simulink model "ScriptDemo"  (R2022b)
settings: configuration reference "TmVcThermal_Configuration_sub" (kept outside this file)
undefined symbols (not defined in the file or in its folder): aaaa, bbbb, cTmComprCtrl_D_u8HvacFlowTable_db, cTmComprCtrl_D_u8HvacFlowTable_sw, cTmComprCtrl_n_i16ChillCmpIMax, cTmComprCtrl_n_i16ChillCmpIMin, cTmComprCtrl_n_i16ChillCmpIMin666, cTmComprCtrl_n_i16ChillCmpPMax, cTmComprCtrl_n_i16ChillCmpPMin, cTmComprCtrl_n_i16CmpChillCoolRpmKiMax, cTmComprCtrl_n_i16CmpChillCoolRpmKiMin, cTmComprCtrl_n_i16CmpChillCoolRpmKpMax, cTmComprCtrl_n_i16CmpChillCoolRpmKpMin, cTmComprCtrl_n_i16CmpCoolRpmKiMax, cTmComprCtrl_n_i16CmpCoolRpmKiMin, cTmComprCtrl_n_i16CmpCoolRpmKpMax, cTmComprCtrl_n_i16CmpCoolRpmKpMin, cTmComprCtrl_n_i16SM4CmpHeatKiMax, cTmComprCtrl_n_i16SM4CmpHeatKiMin, cTmComprCtrl_n_i16SM4CmpHeatKpMax, cTmComprCtrl_n_i16SM4CmpHeatKpMin, cTmComprCtrl_n_i16SM5CmpHeatKiMax, cTmComprCtrl_n_i16SM5CmpHeatKiMin, cTmComprCtrl_n_i16SM5CmpHeatKpMax, cTmComprCtrl_n_i16SM5CmpHeatKpMin, cTmComprCtrl_n_i16SM6CmpHeatKiMax, cTmComprCtrl_n_i16SM6CmpHeatKiMin, cTmComprCtrl_n_i16SM6CmpHeatKpMax, cTmComprCtrl_n_i16SM6CmpHeatKpMin, cTmComprCtrl_n_u16CmpMaxSpdFanFltLimt, cTmComprCtrl_n_u16CmpMaxSpdLoSidePFltLimt, cTmComprCtrl_n_u16CmpMaxSpdSensorFltLimt, cTmComprCtrl_n_u16CompMinRpm, cTmComprCtrl_n_u16CompRpmIncThres, cTmComprCtrl_t_u16BattCooltFFPeriod, cTmComprCtrl_t_u16BattCooltPIPeriod, cTmComprCtrl_t_u16CmpCoolFFPeriod, cTmComprCtrl_t_u16CmpCoolPIPeriod, cTmComprCtrl_t_u16CoolCmpChillFFPeriod, cTmComprCtrl_t_u16CoolCmpChillPIPeriod, cTmComprCtrl_t_u16SM4CmpHeatFFPeriod, cTmComprCtrl_t_u16SM4CmpHeatPIPeriod, cTmComprCtrl_t_u16SM5CmpHeatFFPeriod, cTmComprCtrl_t_u16SM5CmpHeatPIPeriod, cTmComprCtrl_t_u16SM6CmpHeatFFPeriod, cTmComprCtrl_t_u16SM6CmpHeatPIPeriod, cTmComprCtrl_Te_EvapClearInteg, cTmComprCtrl_Te_i16HpReqTempSaturoffset, cTmComprCtrl_Te_i16SatLpReplaceDiff, cTmComprCtrl_Te_i16SM3BatDiffStartEvapDecOffset, cTmComprCtrl_Te_i16SM3EvapLo, cTmComprCtrl_Te_i16SM3TBatDiffEntEvapDecOffset, cTmComprCtrl_Te_i16SM3TBatDiffEntEvapDecOffsetQuit, cTmComprCtrl_Te_s32ErrCmpChillPIContinueCoolH, cTmComprCtrl_Te_s32ErrCmpChillPIContinueCoolL, cTmComprCtrl_Te_s32ErrCmpPIContinueChillH, cTmComprCtrl_Te_s32ErrCmpPIContinueChillL, cTmComprCtrl_Te_s32ErrCmpPIContinueCoolH, cTmComprCtrl_Te_s32ErrCmpPIContinueCoolL, cTmComprCtrl_Te_s32ErrCmpPIContinueHeatH ... (+398)
libraries: simulink x846, PCMULib x711, simulink_need_slupdate x4
(part 29 of 49)

== system ScriptDemo/Create/createMerge/After/SM3SM23/ID26262_SM3FF ==
  note: 0704：这里为什么用误差来查表？
  sTmSigProces_Te_s32EvapFanReqRamp : Inport  OutDataTypeStr=single
  sTmIn_D_u8DCChrgSt : Inport  Port=2  OutDataTypeStr=uint8
  sTmIn_Te_s32BattHv : Inport  Port=3  OutDataTypeStr=single
  sTmIn_X_s32ClimtRcirc : Inport  Port=4  OutDataTypeStr=single
  sTmComprCtrl_D_u8HvacFlowLevel : Inport  Port=5  OutDataTypeStr=uint8
  sTmSigProces_D_u8HvBattCoolgReq : Inport  Port=6  OutDataTypeStr=uint8
  xTmComprCtrl_B_CompOnReqCompOn : Inport  Port=7  OutDataTypeStr=boolean
  sTmIn_D_u8HeatPump : Inport  Port=8  OutDataTypeStr=uint8
  1-D Lookup Table1 : Lookup_n-D  NumberOfTableDimensions=1  BreakpointsForDimension1=tTmComprCtrl_n_s32Kcmp_X  BreakpointsForDimension1DataTypeStr=Inherit: Inherit from 'Breakpoint data'  Table=tTmComprCtrl_n_s32Kcmp  TableDataTypeStr=Inherit: Inherit from 'Table data'  ExtrapMethod=Clip  InternalRulePriority=Speed  OutDataTypeStr=Inherit: Inherit via back propagation  RndMeth=Simplest  InputSameDT=off
  1-D Lookup Table2 : Lookup_n-D  NumberOfTableDimensions=1  BreakpointsForDimension1=tTmComprCtrl_n_s32KChill_X  BreakpointsForDimension1DataTypeStr=Inherit: Inherit from 'Breakpoint data'  Table=tTmComprCtrl_n_s32KChill  TableDataTypeStr=Inherit: Inherit from 'Table data'  ExtrapMethod=Clip  InternalRulePriority=Speed  OutDataTypeStr=Inherit: Inherit via back propagation  RndMeth=Simplest  InputSameDT=off
  Add : Sum  OutDataTypeStr=uint16
  From7 : From  Commented=on  GotoTag=sTmIn_Te_s32HvBattCooltTReq
  Product : Product
  Product1 : Product
  SM1FFEnable : Subsystem
  SM2FFEnable : Subsystem
  SM3SM1FF : Subsystem
  SM3SM2FF : Subsystem
  SM3FF : Outport
  wires:
  [sTmIn_Te_s32BattHv] -> 1-D Lookup Table2/1
  1-D Lookup Table1/1 -> Product1/1  "Kcmp"
  1-D Lookup Table2/1 -> Product/2  "KChill"
  [sTmSigProces_Te_s32TAmb] -> 1-D Lookup Table1/1
  Product/1 -> Add/1
  [SM1FF] -> Product/1
  Product1/1 -> Add/2
  [SM2FF] -> Product1/2
  Add/1 -> SM3FF/1
  ? -> [sTmIn_Te_s32HvBattCooltTReq]
  sTmSigProces_Te_s32EvapFanReqRamp/1 -> [sTmSigProces_Te_s32EvapFanReqRamp]
  sTmIn_D_u8DCChrgSt/1 -> [sTmIn_D_u8DCChrgSt]
  ? -> [sTmSigProces_Te_s32TAmb]
  sTmIn_Te_s32BattHv/1 -> [sTmIn_Te_s32BattHv]
  sTmIn_X_s32ClimtRcirc/1 -> [sTmIn_X_s32ClimtRcirc]
  sTmComprCtrl_D_u8HvacFlowLevel/1 -> [sTmComprCtrl_D_u8HvacFlowLevel]
  sTmSigProces_D_u8HvBattCoolgReq/1 -> [sTmSigProces_D_u8HvBattCoolgReq]
  SM1FFEnable/1(SM1FFEnable_B_SM1FFEnable) -> [SM1FFEnable_B_SM1FFEnable]
  [xTmComprCtrl_B_CompOnReqCompOn] -> SM1FFEnable/1(xTmComprCtrl_B_CompOnReqCompOn)
  [SM1FFEnable_B_SM1FFEnable] -> SM3SM1FF/Enable
  [sTmSigProces_D_u8HvBattCoolgReq] -> SM3SM1FF/2(sTmSigProces_D_u8HvBattCoolgReq)
  [sTmIn_D_u8DCChrgSt] -> SM3SM1FF/1(sTmIn_D_u8DCChrgSt)
  [sTmIn_Te_s32HvBattCooltTReq] -> ?
  [SM2FFEnable_B_SM2FFEnable] -> SM3SM2FF/Enable
  [xTmComprCtrl_B_CompOnReqCompOn] -> SM2FFEnable/1(xTmComprCtrl_B_CompOnReqCompOn)
  SM2FFEnable/1(SM2FFEnable_B_SM2FFEnable) -> [SM2FFEnable_B_SM2FFEnable]
  SM3SM1FF/1(SM1FF) -> [SM1FF]  "rTmComprCtrl_n_u16ComprRpmFFSM3SM1"
  xTmComprCtrl_B_CompOnReqCompOn/1 -> [xTmComprCtrl_B_CompOnReqCompOn]
  [sTmSigProces_Te_s32TAmb] -> ?
  SM3SM2FF/1(SM2FF) -> [SM2FF]  "rTmComprCtrl_n_u16ComprRpmFFSM3SM2"
  [sTmSigProces_Te_s32EvapFanReqRamp] -> SM3SM2FF/1(sTmSigProces_Te_s32EvapFanReqRamp)
  [sTmSigProces_Te_s32TAmb] -> ?
  [sTmIn_X_s32ClimtRcirc] -> SM3SM2FF/2(sTmIn_X_s32ClimtRcirc)
  [sTmComprCtrl_D_u8HvacFlowLevel] -> SM3SM2FF/3(sTmComprCtrl_D_u8HvacFlowLevel)
  [sTmIn_D_u8HeatPump] -> SM3SM2FF/4(sTmIn_D_u8HeatPump)
  sTmIn_D_u8HeatPump/1 -> [sTmIn_D_u8HeatPump]
  [sTmIn_D_u8HeatPump] -> SM3SM1FF/3(sTmIn_D_u8HeatPump)

== system ScriptDemo/Create/createMerge/After/SM3SM23/ID26263_SM3Error ==
  note: 非热泵
  note: 1: 非热泵
      | 2：热泵
  note: 热泵
  sTmSigProces_Te_s32EvapFanReqRamp : Inport  OutDataTypeStr=single
  sTmIn_D_u8HeatPump : Inport  Port=2  OutDataTypeStr=uint8
  sTmSigProces_D_u8HvBattCoolgReq : Inport  Port=3  OutDataTypeStr=uint8
  sTmSigProces_Te_s32EvapFanFilter : Inport  Port=4  OutDataTypeStr=single
  xTmComprCtrl_B_ModeChanged : Inport  Port=5  OutDataTypeStr=boolean
  Compare To Constant1 : simulink/Logic and Bit Operations/Compare To Constant  relop===  const=2  OutDataTypeStr=boolean
  SM3HPErr : Subsystem
  SM3NHPErr : Subsystem
  Switch : Switch  Criteria=u2 ~= 0  SaturateOnIntegerOverflow=off  InputSameDT=off
  rTmComprCtrl_Te_s32TempError : Outport
  wires:
  Compare To Constant1/1 -> Switch/2
  [sTmIn_D_u8HeatPump] -> Compare To Constant1/1
  Switch/1 -> rTmComprCtrl_Te_s32TempError/1
  SM3NHPErr/1(SM3NHPErr_Te_s32Error) -> Switch/3
  SM3HPErr/1(SM3HPErr_Te_s32Error) -> Switch/1
  [sTmSigProces_Te_s32EvapFanReqRamp] -> SM3HPErr/1(sTmSigProces_Te_s32EvapFanReqRamp)
  [sTmIn_Te_s32HvBattCooltTReq] -> ?
  [sTmSigProces_Te_s32EvapFanFilter] -> SM3HPErr/2(sTmSigProces_Te_s32EvapFanFilter)
  [sTmSigProces_Te_s32HvBattCooltTFilter] -> ?
  [sTmSigProces_Te_s32EvapFanReqRamp] -> SM3NHPErr/1(sTmSigProces_Te_s32EvapFanReqRamp)
  [sTmIn_Te_s32HvBattCooltTReq] -> ?
  [sTmSigProces_D_u8HvBattCoolgReq] -> SM3NHPErr/2(sTmSigProces_D_u8HvBattCoolgReq)
  [sTmSigProces_Te_s32EvapFanFilter] -> SM3NHPErr/3(sTmSigProces_Te_s32EvapFanFilter)
  [sTmSigProces_Te_s32HvBattCooltTFilter] -> ?
  sTmSigProces_Te_s32EvapFanReqRamp/1 -> [sTmSigProces_Te_s32EvapFanReqRamp]
  sTmIn_D_u8HeatPump/1 -> [sTmIn_D_u8HeatPump]
  ? -> [sTmIn_Te_s32HvBattCooltTReq]
  sTmSigProces_D_u8HvBattCoolgReq/1 -> [sTmSigProces_D_u8HvBattCoolgReq]
  sTmSigProces_Te_s32EvapFanFilter/1 -> [sTmSigProces_Te_s32EvapFanFilter]
  ? -> [sTmSigProces_Te_s32HvBattCooltTFilter]
  [xTmComprCtrl_B_ModeChanged] -> SM3HPErr/3(xTmComprCtrl_B_ModeChanged)
  xTmComprCtrl_B_ModeChanged/1 -> [xTmComprCtrl_B_ModeChanged]

== system ScriptDemo/Create/createMerge/After/SM3SM23/SM3SM1Error ==
  "NegAndPosCheck " : Subsystem  AncestorBlock=CustomLib/TempNegAndPosCheck
  Terminator : Terminator
  rTmComprCtrl_Te_s32TempError : Outport  OutDataTypeStr=single
  wires:
  ? -> "NegAndPosCheck "/2(Acture)
  "NegAndPosCheck "/2(Dvt_PosFlag) -> Terminator/1
  ? -> "NegAndPosCheck "/1(SetPoint)
  "NegAndPosCheck "/1(Dvt) -> rTmComprCtrl_Te_s32TempError/1

== system ScriptDemo/Create/createMerge/After/SM3SM23/SM3SM2Error ==
  note: 控制对象为低压饱和温度
  note: 控制对象为蒸发器温度滤波值
  sTmSigProces_Te_s32EvapFanReqRamp : Inport  OutDataTypeStr=single
  sTmDiag_D_u8TeEvapFltSt : Inport  Port=2  OutDataTypeStr=uint8
  sTmSigProces_Te_s32EvapFanFilter : Inport  Port=3  OutDataTypeStr=single
  sTmSigProces_Te_s32SatLp : Inport  Port=4  OutDataTypeStr=single
  yTmRefriModeMgr_B_CoolOCRMode : Inport  Port=5  OutDataTypeStr=boolean
  Add : Sum  Inputs=+-  OutDataTypeStr=single
  Compare To Constant : simulink/Logic and Bit Operations/Compare To Constant  relop===  const=1  OutDataTypeStr=boolean
  Constant : Constant  Value=3  OutDataTypeStr=single
  Constant2 : Constant  Value=cTmComprCtrl_Te_i16SatLpReplaceDiff  OutDataTypeStr=int16
  NegAndPosCheck 1 : Subsystem  AncestorBlock=CustomLib/TempNegAndPosCheck
  Saturation1 : Saturate  UpperLimit=12  LowerLimit=3
  Switch1 : Switch  Criteria=u2 ~= 0  SaturateOnIntegerOverflow=off  InputSameDT=off
  Switch2 : Switch  Criteria=u2 ~= 0  SaturateOnIntegerOverflow=off  InputSameDT=off
  Terminator : Terminator
  rTmComprCtrl_Te_s32TempError : Outport
  wires:
  [sTmDiag_D_u8TeEvapFltSt] -> Switch1/2
  [sTmSigProces_Te_s32SatLp] -> Add/1
  Constant2/1 -> Add/2
  Switch2/1 -> Saturation1/1
  NegAndPosCheck 1/2(Dvt_PosFlag) -> Terminator/1
  NegAndPosCheck 1/1(Dvt) -> rTmComprCtrl_Te_s32TempError/1
  Add/1 -> Switch1/1
  Saturation1/1 -> NegAndPosCheck 1/1(SetPoint)
  sTmSigProces_Te_s32EvapFanReqRamp/1 -> [sTmSigProces_Te_s32EvapFanReqRamp]  "sTmSigProces_Te_s32EvapFanReqRamp"
  sTmDiag_D_u8TeEvapFltSt/1 -> [sTmDiag_D_u8TeEvapFltSt]  "sTmDiag_D_u8TeEvapFltSt"
  sTmSigProces_Te_s32EvapFanFilter/1 -> [sTmSigProces_Te_s32EvapFanFilter]  "sTmSigProces_Te_s32EvapFanFilter"
  sTmSigProces_Te_s32SatLp/1 -> [sTmSigProces_Te_s32SatLp]  "sTmSigProces_Te_s32SatLp"
  [yTmRefriModeMgr_B_CoolOCRMode] -> Compare To Constant/1
  Compare To Constant/1 -> Switch2/2
  Constant/1 -> Switch2/1
  yTmRefriModeMgr_B_CoolOCRMode/1 -> [yTmRefriModeMgr_B_CoolOCRMode]  "yTmRefriModeMgr_B_CoolOCRMode"
  [sTmSigProces_Te_s32EvapFanReqRamp] -> Switch2/3
  [sTmSigProces_Te_s32EvapFanFilter] -> Switch1/3
  Switch1/1 -> NegAndPosCheck 1/2(Acture)

== system ScriptDemo/Create/createMerge/After/SM3SM23/SM3_Ki ==
  note: 等级1或2
  note: 等级3
  SM1Error : Inport
  SM2Error : Inport  Port=2
  sTmIn_D_u8DCChrgSt : Inport  Port=3  OutDataTypeStr=uint8
  sTmIn_D_u8HeatPump : Inport  Port=4  OutDataTypeStr=uint8
  sTmIn_X_s32ClimtRcirc : Inport  Port=5  OutDataTypeStr=single
  sTmComprCtrl_D_u8HvacFlowLevel : Inport  Port=6  OutDataTypeStr=uint8
  sTmSigProces_D_u8BattThermReq : Inport  Port=7  OutDataTypeStr=uint8
  sTmSigProces_D_u8HvBattCoolgReq : Inport  Port=8  OutDataTypeStr=uint8
  Add : Sum
  Add1 : Sum
  Compare To Constant : simulink/Logic and Bit Operations/Compare To Constant  relop===  const=3  OutDataTypeStr=boolean
  SM1Ki : Subsystem
  SM2Ki : Subsystem
  SM3SM1LikeKi : Subsystem
  SM3SM2LikeKi : Subsystem
  Switch : Switch  Criteria=u2 ~= 0  SaturateOnIntegerOverflow=off  InputSameDT=off
  Terminator : Terminator
  SM3Ki : Outport
  wires:
  [sTmIn_D_u8DCChrgSt] -> SM1Ki/2(sTmIn_D_u8DCChrgSt)
  [SM1Error] -> SM1Ki/4(Error)
  [sTmSigProces_D_u8HvBattCoolgReq] -> SM1Ki/3(sTmSigProces_D_u8HvBattCoolgReq)
  SM1Ki/1(SM1Ki) -> [SM1Ki]  "rTmComprCtrl_n_u16ComprRpmKiSM3SM1"
  [sTmSigProces_D_u8BattThermReq] -> SM1Ki/1(sTmSigProces_D_u8BattThermReq)
  [sTmComprCtrl_D_u8HvacFlowLevel] -> SM2Ki/3(sTmComprCtrl_D_u8HvacFlowLevel)
  [SM2Error] -> SM2Ki/1(Error)
  [sTmSigProces_Te_s32TAmb] -> ?
  [sTmIn_X_s32ClimtRcirc] -> SM2Ki/2(sTmIn_X_s32ClimtRcirc)
  [sTmIn_X_s32ClimtRcirc] -> SM3SM2LikeKi/2(sTmIn_X_s32ClimtRcirc)
  SM3SM2LikeKi/1(Ki) -> [SM3SM2LikeKi]  "rTmComprCtrl_n_u16ComprRpmKiSM3SM2Like"
  [SM2Error] -> SM3SM2LikeKi/1(Error)
  [sTmSigProces_Te_s32TAmb] -> ?
  [sTmComprCtrl_D_u8HvacFlowLevel] -> SM3SM2LikeKi/3(sTmComprCtrl_D_u8HvacFlowLevel)
  SM3SM1LikeKi/1(Ki) -> [SM3SM1LikeKi]  "rTmComprCtrl_n_u16ComprRpmKiSM3SM1Like"
  [sTmSigProces_D_u8HvBattCoolgReq] -> SM3SM1LikeKi/3(sTmSigProces_D_u8HvBattCoolgReq)
  [sTmSigProces_D_u8BattThermReq] -> SM3SM1LikeKi/1(sTmSigProces_D_u8BattThermReq)
  [SM1Error] -> SM3SM1LikeKi/4(error)
  [sTmIn_D_u8DCChrgSt] -> SM3SM1LikeKi/2(sTmIn_D_u8DCChrgSt)
  SM1Error/1 -> [SM1Error]
  SM2Error/1 -> [SM2Error]
  sTmIn_D_u8DCChrgSt/1 -> [sTmIn_D_u8DCChrgSt]
  sTmIn_D_u8HeatPump/1 -> [sTmIn_D_u8HeatPump]
  ? -> [sTmSigProces_Te_s32TAmb]
  sTmIn_X_s32ClimtRcirc/1 -> [sTmIn_X_s32ClimtRcirc]
  sTmComprCtrl_D_u8HvacFlowLevel/1 -> [sTmComprCtrl_D_u8HvacFlowLevel]
  sTmSigProces_D_u8BattThermReq/1 -> [sTmSigProces_D_u8BattThermReq]
  sTmSigProces_D_u8HvBattCoolgReq/1 -> [sTmSigProces_D_u8HvBattCoolgReq]
  Add/1 -> Switch/3
  [SM3SM1LikeKi] -> Add/2
  [SM2Ki] -> Add/1
  [SM3SM2LikeKi] -> Add1/2
  [SM1Ki] -> Add1/1
  [sTmSigProces_D_u8HvBattCoolgReq] -> Compare To Constant/1
  Compare To Constant/1 -> Switch/2
  Switch/1 -> SM3Ki/1
  [sTmIn_D_u8HeatPump] -> Terminator/1
  Add1/1 -> Switch/1
  SM2Ki/1(SM2Ki) -> [SM2Ki]  "rTmComprCtrl_n_u16ComprRpmKiSM3SM2"

== system ScriptDemo/Create/createMerge/After/SM3SM23/SM3_Kp ==
  note: 等级1或2
  note: 等级3
  SM1Error : Inport
  SM2Error : Inport  Port=2
  sTmIn_D_u8DCChrgSt : Inport  Port=3  OutDataTypeStr=uint8
  sTmIn_D_u8HeatPump : Inport  Port=4  OutDataTypeStr=uint8
  sTmIn_X_s32ClimtRcirc : Inport  Port=5  OutDataTypeStr=single
  sTmComprCtrl_D_u8HvacFlowLevel : Inport  Port=6  OutDataTypeStr=uint8
  sTmSigProces_D_u8BattThermReq : Inport  Port=7  OutDataTypeStr=uint8
  sTmSigProces_D_u8HvBattCoolgReq : Inport  Port=8  OutDataTypeStr=uint8
  Add : Sum
  Add1 : Sum
  Compare To Constant : simulink/Logic and Bit Operations/Compare To Constant  relop===  const=3  OutDataTypeStr=boolean
  SM1Kp : Subsystem
  SM2Kp : Subsystem
  SM3SM1LikeKp : Subsystem
  SM3SM2LikeKp : Subsystem
  Switch : Switch  Criteria=u2 ~= 0  SaturateOnIntegerOverflow=off  InputSameDT=off
  Terminator : Terminator
  SM3Kp : Outport
  wires:
  [SM1Error] -> SM3SM1LikeKp/4(error)
  Switch/1 -> SM3Kp/1
  SM1Kp/1(SM1Kp) -> [SM1Kp]  "rTmComprCtrl_n_u16ComprRpmKpSM3SM1"
  [SM1Error] -> SM1Kp/4(Error)
  [sTmIn_D_u8DCChrgSt] -> SM1Kp/2(sTmIn_D_u8DCChrgSt)
  [sTmSigProces_D_u8HvBattCoolgReq] -> SM1Kp/3(sTmSigProces_D_u8HvBattCoolgReq)
  [sTmSigProces_D_u8BattThermReq] -> SM1Kp/1(sTmSigProces_D_u8BattThermReq)
  [SM2Error] -> SM2Kp/1(Error)
  [sTmComprCtrl_D_u8HvacFlowLevel] -> SM2Kp/3(sTmComprCtrl_D_u8HvacFlowLevel)
  [sTmIn_X_s32ClimtRcirc] -> SM2Kp/2(sTmIn_X_s32ClimtRcirc)
  [sTmSigProces_Te_s32TAmb] -> ?
  SM3SM1LikeKp/1(Kp) -> [SM3SM1LikeKp]  "rTmComprCtrl_n_u16ComprRpmKpSM3SM1Like"
  [sTmSigProces_D_u8BattThermReq] -> SM3SM1LikeKp/1(sTmSigProces_D_u8BattThermReq)
  [sTmIn_D_u8DCChrgSt] -> SM3SM1LikeKp/2(sTmIn_D_u8DCChrgSt)
  [sTmSigProces_D_u8HvBattCoolgReq] -> SM3SM1LikeKp/3(sTmSigProces_D_u8HvBattCoolgReq)
  [SM2Kp] -> Add/1
  [SM3SM1LikeKp] -> Add/2
  SM1Error/1 -> [SM1Error]
  SM2Error/1 -> [SM2Error]
  sTmIn_D_u8DCChrgSt/1 -> [sTmIn_D_u8DCChrgSt]
  sTmIn_D_u8HeatPump/1 -> [sTmIn_D_u8HeatPump]
  ? -> [sTmSigProces_Te_s32TAmb]
  sTmIn_X_s32ClimtRcirc/1 -> [sTmIn_X_s32ClimtRcirc]
  sTmComprCtrl_D_u8HvacFlowLevel/1 -> [sTmComprCtrl_D_u8HvacFlowLevel]
  sTmSigProces_D_u8BattThermReq/1 -> [sTmSigProces_D_u8BattThermReq]
  sTmSigProces_D_u8HvBattCoolgReq/1 -> [sTmSigProces_D_u8HvBattCoolgReq]
  [sTmIn_X_s32ClimtRcirc] -> SM3SM2LikeKp/2(sTmIn_X_s32ClimtRcirc)
  [sTmComprCtrl_D_u8HvacFlowLevel] -> SM3SM2LikeKp/3(sTmComprCtrl_D_u8HvacFlowLevel)
  [SM2Error] -> SM3SM2LikeKp/1(Error)
  [sTmSigProces_Te_s32TAmb] -> ?
  SM3SM2LikeKp/1(Kp) -> [SM3SM2LikeKp]  "rTmComprCtrl_n_u16ComprRpmKpSM3SM2Like"
  [sTmSigProces_D_u8HvBattCoolgReq] -> Compare To Constant/1
  [sTmIn_D_u8HeatPump] -> Terminator/1
  Compare To Constant/1 -> Switch/2
  [SM3SM2LikeKp] -> Add1/2
  [SM1Kp] -> Add1/1
  Add1/1 -> Switch/1
  Add/1 -> Switch/3
  SM2Kp/1(SM2Kp) -> [SM2Kp]  "rTmComprCtrl_n_u16ComprRpmKpSM3SM2"

== system ScriptDemo/Create/createMerge/After/SM4/ID26259_SM4Error ==
  note: 制冷是实际-请求
      | 这里制热是请求-实际
  note: 未实现
      | 暖风芯体背风温度目标值∈[30, 60] ℃ 。
  note: 无PTC补热
  note: PTC 补热模式
  sTmSigProces_Te_s32SatHp : Inport
  yTmHvchCtrl_B_HpcPtcEnad : Inport  Port=2
  sTmSigProces_Te_s32HeatrAirTReqRamp : Inport  Port=3
  sTmSigProces_Te_s32HvacHexAirTFilter : Inport  Port=4
  Add2 : Sum
  Constant5 : Constant  Value=cTmComprCtrl_Te_i16HpReqTempSaturoffset
  NegAndPosCheck 4 : Subsystem  AncestorBlock=CustomLib/TempNegAndPosCheck
  NegAndPosCheck 5 : Subsystem  AncestorBlock=CustomLib/TempNegAndPosCheck
  Saturation3 : Saturate  UpperLimit=70  LowerLimit=15
  Switch2 : Switch  Criteria=u2 ~= 0  SaturateOnIntegerOverflow=off  InputSameDT=off
  Terminator : Terminator
  Terminator1 : Terminator
  Unary Minus : UnaryMinus
  rTmComprCtrl_Te_s32TempError : Outport
  wires:
  sTmSigProces_Te_s32SatHp/1 -> NegAndPosCheck 4/2(Acture)
  NegAndPosCheck 5/1(Dvt) -> Switch2/3
  sTmSigProces_Te_s32HeatrAirTReqRamp/1 -> Saturation3/1
  Switch2/1 -> Unary Minus/1
  NegAndPosCheck 5/2(Dvt_PosFlag) -> Terminator/1
  NegAndPosCheck 4/1(Dvt) -> Switch2/1
  Constant5/1 -> Add2/1
  NegAndPosCheck 4/2(Dvt_PosFlag) -> Terminator1/1
  sTmSigProces_Te_s32HvacHexAirTFilter/1 -> NegAndPosCheck 5/2(Acture)
  yTmHvchCtrl_B_HpcPtcEnad/1 -> Switch2/2
  Saturation3/1 -> Add2/2, NegAndPosCheck 5/1(SetPoint)
  Add2/1 -> NegAndPosCheck 4/1(SetPoint)
  Unary Minus/1 -> rTmComprCtrl_Te_s32TempError/1

== system ScriptDemo/Create/createMerge/After/SM4/ID26297_SM4FF ==
  sTmComprCtrl_D_u8HvacFlowLevel : Inport  OutDataTypeStr=uint8
  sTmSigProces_Te_s32HeatrAirTReqRamp : Inport  Port=2
  Enable : EnablePort
  1-D Lookup Table : Lookup_n-D  NumberOfTableDimensions=1  BreakpointsForDimension1=tTmComprCtrl_fac_s32FFSM4CompHeatAmbFactor_X  BreakpointsForDimension1DataTypeStr=Inherit: Inherit from 'Breakpoint data'  Table=tTmComprCtrl_fac_s32FFSM4CompHeatAmbFactor  TableDataTypeStr=Inherit: Inherit from 'Table data'  ExtrapMethod=Clip  InternalRulePriority=Speed  OutDataTypeStr=Inherit: Inherit via back propagation  RndMeth=Simplest  InputSameDT=off
  Flow2Rpm : Subsystem  mask{BlwHeatLevel_db=cTmComprCtrl_D_u8HvacFlowTable_db, BlwHeatLevel_sw=cTmComprCtrl_D_u8HvacFlowTable_sw, FFBlw1=mTmComprCtrl_n_u16FFSM4CompHeatRpm_Flow1, FFBlw1_Y=mTmComprCtrl_n_u16FFSM4CompHeatRpm_Flow1_Y, FFBlw1_X=mTmComprCtrl_n_u16FFSM4CompHeatRpm_Flow1_X, FFBlw3=mTmComprCtrl_n_u16FFSM4CompHeatRpm_Flow3, FFBlw3_Y=mTmComprCtrl_n_u16FFSM4CompHeatRpm_Flow3_Y, FFBlw3_X=mTmComprCtrl_n_u16FFSM4CompHeatRpm_Flow3_X, FFBlw5=mTmComprCtrl_n_u16FFSM4CompHeatRpm_Flow5, FFBlw5_Y=mTmComprCtrl_n_u16FFSM4CompHeatRpm_Flow5_Y, FFBlw5_X=mTmComprCtrl_n_u16FFSM4CompHeatRpm_Flow5_X, FFBlw7=mTmComprCtrl_n_u16FFSM4CompHeatRpm_Flow7, FFBlw7_Y=mTmComprCtrl_n_u16FFSM4CompHeatRpm_Flow7_Y, FFBlw7_X=mTmComprCtrl_n_u16FFSM4CompHeatRpm_Flow7_X, FFBlw9=mTmComprCtrl_n_u16FFSM4CompHeatRpm_Flow9, FFBlw9_Y=mTmComprCtrl_n_u16FFSM4CompHeatRpm_Flow9_Y, FFBlw9_X=mTmComprCtrl_n_u16FFSM4CompHeatRpm_Flow9_X}
      mask DialogControl ParameterGroupVar Prompt: 参数
  Product : Product  OutDataTypeStr=uint16
  SM4FF : Outport
  wires:
  sTmComprCtrl_D_u8HvacFlowLevel/1 -> Flow2Rpm/1(md_u8Blw)
  ? -> Flow2Rpm/2(breakpoint1)
  sTmSigProces_Te_s32HeatrAirTReqRamp/1 -> Flow2Rpm/3(breakpoint2)
  [sTmSigProces_Te_s32TAmb] -> 1-D Lookup Table/1
  1-D Lookup Table/1 -> Product/2  "rTmComprCtrl_fac_s32FFSM4CompHeatAmbFactor"
  Flow2Rpm/1(Flow2Rpm) -> Product/1  "rTmComprCtrl_n_u16FFSM4CompHeatRpm"
  Product/1 -> SM4FF/1
  ? -> [sTmSigProces_Te_s32TAmb]

== system ScriptDemo/Create/createMerge/After/SM4/SM24FFEnable ==
  xTmComprCtrl_B_CompOnReqCompOn : Inport  OutDataTypeStr=boolean
  Compare To Constant2 : simulink/Logic and Bit Operations/Compare To Constant  relop===  const=0  OutDataTypeStr=boolean
  Compare To Constant3 : simulink/Logic and Bit Operations/Compare To Constant  relop===  const=1  OutDataTypeStr=boolean
  Logical Operator3 : Logic  AllPortsSameDT=off  OutDataTypeStr=boolean
  PeriodTrig : Subsystem  mask{CounterLim=cTmComprCtrl_t_u16SM4CmpHeatFFPeriod}
      mask DialogControl ParameterGroupVar Prompt: 参数
  Unit Delay : UnitDelay  SampleTime=-1  HasFrameUpgradeWarning=on
  SM4FFEnable_B_SM4FFEnable : Outport  OutDataTypeStr=boolean
  wires:
  Unit Delay/1 -> Compare To Constant2/1
  [xTmComprCtrl_B_CompOnReqCompOn] -> Compare To Constant3/1, Unit Delay/1
  Compare To Constant2/1 -> Logical Operator3/1
  Logical Operator3/1 -> PeriodTrig/1(Counter_Reset)
  Compare To Constant3/1 -> Logical Operator3/2
  xTmComprCtrl_B_CompOnReqCompOn/1 -> [xTmComprCtrl_B_CompOnReqCompOn]
  PeriodTrig/1(Counter_Trig) -> SM4FFEnable_B_SM4FFEnable/1

== system ScriptDemo/Create/createMerge/After/SM4/SM4_Ki ==
  sTmComprCtrl_D_u8HvacFlowLevel : Inport  OutDataTypeStr=uint8
  rTmComprCtrl_Te_s32TempError : Inport  Port=2
  Flow2Rpm : Subsystem  mask{BlwHeatLevel_db=cTmComprCtrl_D_u8HvacFlowTable_db, BlwHeatLevel_sw=cTmComprCtrl_D_u8HvacFlowTable_sw, FFBlw1=mTmComprCtrl_n_u16KiSM4CompHeatRpm_Flow1, FFBlw1_Y=mTmComprCtrl_n_u16KiSM4CompHeatRpm_Flow1_Y, FFBlw1_X=mTmComprCtrl_n_u16KiSM4CompHeatRpm_Flow1_X, FFBlw3=mTmComprCtrl_n_u16KiSM4CompHeatRpm_Flow3, FFBlw3_Y=mTmComprCtrl_n_u16KiSM4CompHeatRpm_Flow3_Y, FFBlw3_X=mTmComprCtrl_n_u16KiSM4CompHeatRpm_Flow3_X, FFBlw5=mTmComprCtrl_n_u16KiSM4CompHeatRpm_Flow5, FFBlw5_Y=mTmComprCtrl_n_u16KiSM4CompHeatRpm_Flow5_Y, FFBlw5_X=mTmComprCtrl_n_u16KiSM4CompHeatRpm_Flow5_X, FFBlw7=mTmComprCtrl_n_u16KiSM4CompHeatRpm_Flow7, FFBlw7_Y=mTmComprCtrl_n_u16KiSM4CompHeatRpm_Flow7_Y, FFBlw7_X=mTmComprCtrl_n_u16KiSM4CompHeatRpm_Flow7_X, FFBlw9=mTmComprCtrl_n_u16KiSM4CompHeatRpm_Flow9, FFBlw9_Y=mTmComprCtrl_n_u16KiSM4CompHeatRpm_Flow9_Y, FFBlw9_X=mTmComprCtrl_n_u16KiSM4CompHeatRpm_Flow9_X}
      mask DialogControl ParameterGroupVar Prompt: 参数
  SM4Ki : Outport
  wires:
  Flow2Rpm/1(Flow2Rpm) -> SM4Ki/1  "mask"
  sTmComprCtrl_D_u8HvacFlowLevel/1 -> Flow2Rpm/1(md_u8Blw)
  ? -> Flow2Rpm/2(breakpoint1)
  rTmComprCtrl_Te_s32TempError/1 -> Flow2Rpm/3(breakpoint2)

== system ScriptDemo/Create/createMerge/After/SM4/SM4_Kp ==
  sTmComprCtrl_D_u8HvacFlowLevel : Inport  OutDataTypeStr=uint8
  rTmComprCtrl_Te_s32TempError : Inport  Port=2
  Flow2Rpm : Subsystem  mask{BlwHeatLevel_db=cTmComprCtrl_D_u8HvacFlowTable_db, BlwHeatLevel_sw=cTmComprCtrl_D_u8HvacFlowTable_sw, FFBlw1=mTmComprCtrl_n_u16KpSM4CompHeatRpm_Flow1, FFBlw1_Y=mTmComprCtrl_n_u16KpSM4CompHeatRpm_Flow1_Y, FFBlw1_X=mTmComprCtrl_n_u16KpSM4CompHeatRpm_Flow1_X, FFBlw3=mTmComprCtrl_n_u16KpSM4CompHeatRpm_Flow3, FFBlw3_Y=mTmComprCtrl_n_u16KpSM4CompHeatRpm_Flow3_Y, FFBlw3_X=mTmComprCtrl_n_u16KpSM4CompHeatRpm_Flow3_X, FFBlw5=mTmComprCtrl_n_u16KpSM4CompHeatRpm_Flow5, FFBlw5_Y=mTmComprCtrl_n_u16KpSM4CompHeatRpm_Flow5_Y, FFBlw5_X=mTmComprCtrl_n_u16KpSM4CompHeatRpm_Flow5_X, FFBlw7=mTmComprCtrl_n_u16KpSM4CompHeatRpm_Flow7, FFBlw7_Y=mTmComprCtrl_n_u16KpSM4CompHeatRpm_Flow7_Y, FFBlw7_X=mTmComprCtrl_n_u16KpSM4CompHeatRpm_Flow7_X, FFBlw9=mTmComprCtrl_n_u16KpSM4CompHeatRpm_Flow9, FFBlw9_Y=mTmComprCtrl_n_u16KpSM4CompHeatRpm_Flow9_Y, FFBlw9_X=mTmComprCtrl_n_u16KpSM4CompHeatRpm_Flow9_X}
      mask DialogControl ParameterGroupVar Prompt: 参数
  SM4Kp : Outport
  wires:
  Flow2Rpm/1(Flow2Rpm) -> SM4Kp/1  "mask"
  sTmComprCtrl_D_u8HvacFlowLevel/1 -> Flow2Rpm/1(md_u8Blw)
  ? -> Flow2Rpm/2(breakpoint1)
  rTmComprCtrl_Te_s32TempError/1 -> Flow2Rpm/3(breakpoint2)

== system ScriptDemo/Create/createMerge/After/SM5/ID26291_SM5FF ==
  note: SM5前馈值
  note: SM5前馈值修正系数
  sTmComprCtrl_D_u8HvacFlowLevel : Inport  OutDataTypeStr=uint8
  sTmSigProces_Te_s32HeatrAirTReqRamp : Inport  Port=2
  sTmSigProces_Te_s32SatLp : Inport  Port=3
  Enable : EnablePort
  2-D Lookup Table5 : Lookup_n-D  NumberOfTableDimensions=1  BreakpointsForDimension1=tTmComprCtrl_fac_s32FFSM5CompHeatBattCooltTFactor_X  BreakpointsForDimension2=mTmComprCtrl_n_u16FFSM5CompHeatRpmOffset_X  BreakpointsForDimension1DataTypeStr=Inherit: Inherit from 'Breakpoint data'  BreakpointsForDimension2DataTypeStr=Inherit: Inherit from 'Breakpoint data'  Table=tTmComprCtrl_fac_s32FFSM5CompHeatBattCooltTFactor  TableDataTypeStr=Inherit: Inherit from 'Table data'  ExtrapMethod=Clip  InternalRulePriority=Speed  OutDataTypeStr=Inherit: Inherit via back propagation  RndMeth=Simplest  InputSameDT=off
  Data Type Conversion : DataTypeConversion  OutDataTypeStr=uint16  SaturateOnIntegerOverflow=off  RndMeth=Floor
  Flow2Rpm : Subsystem  mask{BlwHeatLevel_db=cTmComprCtrl_D_u8HvacFlowTable_db, BlwHeatLevel_sw=cTmComprCtrl_D_u8HvacFlowTable_sw, FFBlw1=mTmComprCtrl_n_u16FFSM5CompHeatRpm_Flow1, FFBlw1_Y=mTmComprCtrl_n_u16FFSM5CompHeatRpm_Flow1_Y, FFBlw1_X=mTmComprCtrl_n_u16FFSM5CompHeatRpm_Flow1_X, FFBlw3=mTmComprCtrl_n_u16FFSM5CompHeatRpm_Flow3, FFBlw3_Y=mTmComprCtrl_n_u16FFSM5CompHeatRpm_Flow3_Y, FFBlw3_X=mTmComprCtrl_n_u16FFSM5CompHeatRpm_Flow3_X, FFBlw5=mTmComprCtrl_n_u16FFSM5CompHeatRpm_Flow5, FFBlw5_Y=mTmComprCtrl_n_u16FFSM5CompHeatRpm_Flow5_Y, FFBlw5_X=mTmComprCtrl_n_u16FFSM5CompHeatRpm_Flow5_X, FFBlw7=mTmComprCtrl_n_u16FFSM5CompHeatRpm_Flow7, FFBlw7_Y=mTmComprCtrl_n_u16FFSM5CompHeatRpm_Flow7_Y, FFBlw7_X=mTmComprCtrl_n_u16FFSM5CompHeatRpm_Flow7_X, FFBlw9=mTmComprCtrl_n_u16FFSM5CompHeatRpm_Flow9, FFBlw9_Y=mTmComprCtrl_n_u16FFSM5CompHeatRpm_Flow9_Y, FFBlw9_X=mTmComprCtrl_n_u16FFSM5CompHeatRpm_Flow9_X}
      mask DialogControl ParameterGroupVar Prompt: 参数
  Product : Product  OutDataTypeStr=uint16
  SM5FF : Outport
  wires:
  sTmSigProces_Te_s32SatLp/1 -> 2-D Lookup Table5/1
  2-D Lookup Table5/1 -> Product/2  "rTmComprCtrl_fac_s32FFSM5CompHeatBattCooltTFactor"
  Product/1 -> SM5FF/1
  sTmComprCtrl_D_u8HvacFlowLevel/1 -> Flow2Rpm/1(md_u8Blw)
  ? -> Flow2Rpm/2(breakpoint1)
  sTmSigProces_Te_s32HeatrAirTReqRamp/1 -> Flow2Rpm/3(breakpoint2)
  Flow2Rpm/1(Flow2Rpm) -> Data Type Conversion/1
  Data Type Conversion/1 -> Product/1  "rTmComprCtrl_n_u16FFSM5CompHeatRpm"

== system ScriptDemo/Create/createMerge/After/SM5/ID26293_SM5Error ==
  note: 未实现
      | 暖风芯体背风温度目标值∈[30, 60] ℃ 。
  note: 无PTC补热
  note: PTC 补热模式
  sTmSigProces_Te_s32SatHp : Inport
  yTmHvchCtrl_B_HpcPtcEnad : Inport  Port=2
  sTmSigProces_Te_s32HeatrAirTReqRamp : Inport  Port=3
  sTmSigProces_Te_s32HvacHexAirTFilter : Inport  Port=4
  Add2 : Sum
  Constant5 : Constant  Value=cTmComprCtrl_Te_i16HpReqTempSaturoffset
  NegAndPosCheck 4 : Subsystem  AncestorBlock=CustomLib/TempNegAndPosCheck
  NegAndPosCheck 5 : Subsystem  AncestorBlock=CustomLib/TempNegAndPosCheck
  Saturation3 : Saturate  UpperLimit=70  LowerLimit=15
  Switch2 : Switch  Criteria=u2 ~= 0  SaturateOnIntegerOverflow=off  InputSameDT=off
  Terminator : Terminator
  Terminator1 : Terminator
  Unary Minus : UnaryMinus
  rTmComprCtrl_Te_s32TempError : Outport
  wires:
  sTmSigProces_Te_s32SatHp/1 -> NegAndPosCheck 4/2(Acture)
  NegAndPosCheck 5/1(Dvt) -> Switch2/3
  sTmSigProces_Te_s32HeatrAirTReqRamp/1 -> Saturation3/1
  Switch2/1 -> Unary Minus/1
  NegAndPosCheck 5/2(Dvt_PosFlag) -> Terminator/1
  NegAndPosCheck 4/1(Dvt) -> Switch2/1
  Constant5/1 -> Add2/1
  NegAndPosCheck 4/2(Dvt_PosFlag) -> Terminator1/1
  sTmSigProces_Te_s32HvacHexAirTFilter/1 -> NegAndPosCheck 5/2(Acture)
  yTmHvchCtrl_B_HpcPtcEnad/1 -> Switch2/2
  Saturation3/1 -> NegAndPosCheck 5/1(SetPoint), Add2/2
  Add2/1 -> NegAndPosCheck 4/1(SetPoint)
  Unary Minus/1 -> rTmComprCtrl_Te_s32TempError/1

== system ScriptDemo/Create/createMerge/After/SM5/SM5FFEnable ==
  xTmComprCtrl_B_CompOnReqCompOn : Inport  OutDataTypeStr=boolean
  Compare To Constant2 : simulink/Logic and Bit Operations/Compare To Constant  relop===  const=0  OutDataTypeStr=boolean
  Compare To Constant3 : simulink/Logic and Bit Operations/Compare To Constant  relop===  const=1  OutDataTypeStr=boolean
  Logical Operator3 : Logic  AllPortsSameDT=off  OutDataTypeStr=boolean
  PeriodTrig : Subsystem  mask{CounterLim=cTmComprCtrl_t_u16SM5CmpHeatFFPeriod}
      mask DialogControl ParameterGroupVar Prompt: 参数
  Unit Delay : UnitDelay  SampleTime=-1  HasFrameUpgradeWarning=on
  SM5FFEnable_B_SM5FFEnable : Outport  OutDataTypeStr=boolean
  wires:
  Unit Delay/1 -> Compare To Constant2/1
  [xTmComprCtrl_B_CompOnReqCompOn] -> Compare To Constant3/1, Unit Delay/1
  Compare To Constant2/1 -> Logical Operator3/1
  Logical Operator3/1 -> PeriodTrig/1(Counter_Reset)
  Compare To Constant3/1 -> Logical Operator3/2
  xTmComprCtrl_B_CompOnReqCompOn/1 -> [xTmComprCtrl_B_CompOnReqCompOn]
  PeriodTrig/1(Counter_Trig) -> SM5FFEnable_B_SM5FFEnable/1

== system ScriptDemo/Create/createMerge/After/SM5/SM5_Ki ==
  sTmComprCtrl_D_u8HvacFlowLevel : Inport  OutDataTypeStr=uint8
  sTmSigProces_Te_s32SatLp : Inport  Port=2
  rTmComprCtrl_Te_s32TempError : Inport  Port=3
  Data Type Conversion : DataTypeConversion  OutDataTypeStr=uint16  SaturateOnIntegerOverflow=off  RndMeth=Floor
  Flow2Rpm : Subsystem  mask{BlwHeatLevel_db=cTmComprCtrl_D_u8HvacFlowTable_db, BlwHeatLevel_sw=cTmComprCtrl_D_u8HvacFlowTable_sw, FFBlw1=mTmComprCtrl_n_u16KiSM5CompHeatRpm_Flow1, FFBlw1_Y=mTmComprCtrl_n_u16KiSM5CompHeatRpm_Flow1_Y, FFBlw1_X=mTmComprCtrl_n_u16KiSM5CompHeatRpm_Flow1_X, FFBlw3=mTmComprCtrl_n_u16KiSM5CompHeatRpm_Flow3, FFBlw3_Y=mTmComprCtrl_n_u16KiSM5CompHeatRpm_Flow3_Y, FFBlw3_X=mTmComprCtrl_n_u16KiSM5CompHeatRpm_Flow3_X, FFBlw5=mTmComprCtrl_n_u16KiSM5CompHeatRpm_Flow5, FFBlw5_Y=mTmComprCtrl_n_u16KiSM5CompHeatRpm_Flow5_Y, FFBlw5_X=mTmComprCtrl_n_u16KiSM5CompHeatRpm_Flow5_X, FFBlw7=mTmComprCtrl_n_u16KiSM5CompHeatRpm_Flow7, FFBlw7_Y=mTmComprCtrl_n_u16KiSM5CompHeatRpm_Flow7_Y, FFBlw7_X=mTmComprCtrl_n_u16KiSM5CompHeatRpm_Flow7_X, FFBlw9=mTmComprCtrl_n_u16KiSM5CompHeatRpm_Flow9, FFBlw9_Y=mTmComprCtrl_n_u16KiSM5CompHeatRpm_Flow9_Y, FFBlw9_X=mTmComprCtrl_n_u16KiSM5CompHeatRpm_Flow9_X}
      mask DialogControl ParameterGroupVar Prompt: 参数
  SM5Ki : Outport
  wires:
  Flow2Rpm/1(Flow2Rpm) -> Data Type Conversion/1
  Data Type Conversion/1 -> SM5Ki/1
  sTmComprCtrl_D_u8HvacFlowLevel/1 -> Flow2Rpm/1(md_u8Blw)
  sTmSigProces_Te_s32SatLp/1 -> Flow2Rpm/2(breakpoint1)
  rTmComprCtrl_Te_s32TempError/1 -> Flow2Rpm/3(breakpoint2)

== system ScriptDemo/Create/createMerge/After/SM5/SM5_Kp ==
  sTmComprCtrl_D_u8HvacFlowLevel : Inport  OutDataTypeStr=uint8
  sTmSigProces_Te_s32SatLp : Inport  Port=2
  rTmComprCtrl_Te_s32TempError : Inport  Port=3
  Data Type Conversion : DataTypeConversion  OutDataTypeStr=uint16  SaturateOnIntegerOverflow=off  RndMeth=Floor
  Flow2Rpm : Subsystem  mask{BlwHeatLevel_db=cTmComprCtrl_D_u8HvacFlowTable_db, BlwHeatLevel_sw=cTmComprCtrl_D_u8HvacFlowTable_sw, FFBlw1=mTmComprCtrl_n_u16KpSM5CompHeatRpm_Flow1, FFBlw1_Y=mTmComprCtrl_n_u16KpSM5CompHeatRpm_Flow1_Y, FFBlw1_X=mTmComprCtrl_n_u16KpSM5CompHeatRpm_Flow1_X, FFBlw3=mTmComprCtrl_n_u16KpSM5CompHeatRpm_Flow3, FFBlw3_Y=mTmComprCtrl_n_u16KpSM5CompHeatRpm_Flow3_Y, FFBlw3_X=mTmComprCtrl_n_u16KpSM5CompHeatRpm_Flow3_X, FFBlw5=mTmComprCtrl_n_u16KpSM5CompHeatRpm_Flow5, FFBlw5_Y=mTmComprCtrl_n_u16KpSM5CompHeatRpm_Flow5_Y, FFBlw5_X=mTmComprCtrl_n_u16KpSM5CompHeatRpm_Flow5_X, FFBlw7=mTmComprCtrl_n_u16KpSM5CompHeatRpm_Flow7, FFBlw7_Y=mTmComprCtrl_n_u16KpSM5CompHeatRpm_Flow7_Y, FFBlw7_X=mTmComprCtrl_n_u16KpSM5CompHeatRpm_Flow7_X, FFBlw9=mTmComprCtrl_n_u16KpSM5CompHeatRpm_Flow9, FFBlw9_Y=mTmComprCtrl_n_u16KpSM5CompHeatRpm_Flow9_Y, FFBlw9_X=mTmComprCtrl_n_u16KpSM5CompHeatRpm_Flow9_X}
      mask DialogControl ParameterGroupVar Prompt: 参数
  SM5Kp : Outport
  wires:
  Flow2Rpm/1(Flow2Rpm) -> Data Type Conversion/1
  Data Type Conversion/1 -> SM5Kp/1
  sTmSigProces_Te_s32SatLp/1 -> Flow2Rpm/2(breakpoint1)
  rTmComprCtrl_Te_s32TempError/1 -> Flow2Rpm/3(breakpoint2)
  sTmComprCtrl_D_u8HvacFlowLevel/1 -> Flow2Rpm/1(md_u8Blw)

== system ScriptDemo/Create/createMerge/After/SM6/ID26282_SM6FF ==
  note: TODO: 这里需要确认下需求
  sTmComprCtrl_D_u8HvacFlowLevel : Inport  OutDataTypeStr=uint8
  sTmSigProces_Te_s32HeatrAirTReqRamp : Inport  Port=2
  Enable : EnablePort
  Flow2Rpm : Subsystem  mask{BlwHeatLevel_db=cTmComprCtrl_D_u8HvacFlowTable_db, BlwHeatLevel_sw=cTmComprCtrl_D_u8HvacFlowTable_sw, FFBlw1=mTmComprCtrl_n_u16FFSM6CompHeatRpm_Flow1, FFBlw1_Y=mTmComprCtrl_n_u16FFSM6CompHeatRpm_Flow1_Y, FFBlw1_X=mTmComprCtrl_n_u16FFSM6CompHeatRpm_Flow1_X, FFBlw3=mTmComprCtrl_n_u16FFSM6CompHeatRpm_Flow3, FFBlw3_Y=mTmComprCtrl_n_u16FFSM6CompHeatRpm_Flow3_Y, FFBlw3_X=mTmComprCtrl_n_u16FFSM6CompHeatRpm_Flow3_X, FFBlw5=mTmComprCtrl_n_u16FFSM6CompHeatRpm_Flow5, FFBlw5_Y=mTmComprCtrl_n_u16FFSM6CompHeatRpm_Flow5_Y, FFBlw5_X=mTmComprCtrl_n_u16FFSM6CompHeatRpm_Flow5_X, FFBlw7=mTmComprCtrl_n_u16FFSM6CompHeatRpm_Flow7, FFBlw7_Y=mTmComprCtrl_n_u16FFSM6CompHeatRpm_Flow7_Y, FFBlw7_X=mTmComprCtrl_n_u16FFSM6CompHeatRpm_Flow7_X, FFBlw9=mTmComprCtrl_n_u16FFSM6CompHeatRpm_Flow9, FFBlw9_Y=mTmComprCtrl_n_u16FFSM6CompHeatRpm_Flow9_Y, FFBlw9_X=mTmComprCtrl_n_u16FFSM6CompHeatRpm_Flow9_X}
      mask DialogControl ParameterGroupVar Prompt: 参数
  SM6FF : Outport
  wires:
  Flow2Rpm/1(Flow2Rpm) -> SM6FF/1
  sTmComprCtrl_D_u8HvacFlowLevel/1 -> Flow2Rpm/1(md_u8Blw)
  sTmSigProces_Te_s32HeatrAirTReqRamp/1 -> Flow2Rpm/3(breakpoint2)
  ? -> Flow2Rpm/2(breakpoint1)

== system ScriptDemo/Create/createMerge/After/SM6/ID26284_SM6Error ==
  note: 暖风芯体背风温度目标值∈[0, 80] ℃ 。
  note: 无PTC补热
  note: PTC 补热模式
  sTmSigProces_Te_s32SatHp : Inport
  yTmHvchCtrl_B_HpcPtcEnad : Inport  Port=2
  sTmSigProces_Te_s32HeatrAirTReqRamp : Inport  Port=3
  sTmSigProces_Te_s32HvacHexAirTFilter : Inport  Port=4
  Add2 : Sum
  Constant5 : Constant  Value=cTmComprCtrl_Te_i16HpReqTempSaturoffset
  NegAndPosCheck 4 : Subsystem  AncestorBlock=CustomLib/TempNegAndPosCheck
  NegAndPosCheck 5 : Subsystem  AncestorBlock=CustomLib/TempNegAndPosCheck
  Saturation2 : Saturate  UpperLimit=70  LowerLimit=15
  Switch2 : Switch  Criteria=u2 ~= 0  SaturateOnIntegerOverflow=off  InputSameDT=off
  Terminator : Terminator
  Terminator1 : Terminator
  Unary Minus : UnaryMinus
  rTmComprCtrl_Te_s32TempError : Outport
  wires:
  sTmSigProces_Te_s32SatHp/1 -> NegAndPosCheck 4/2(Acture)
  NegAndPosCheck 5/1(Dvt) -> Switch2/3
  sTmSigProces_Te_s32HeatrAirTReqRamp/1 -> Saturation2/1
  Switch2/1 -> Unary Minus/1
  NegAndPosCheck 5/2(Dvt_PosFlag) -> Terminator/1
  NegAndPosCheck 4/1(Dvt) -> Switch2/1
  Constant5/1 -> Add2/1
  NegAndPosCheck 4/2(Dvt_PosFlag) -> Terminator1/1
  sTmSigProces_Te_s32HvacHexAirTFilter/1 -> NegAndPosCheck 5/2(Acture)
  yTmHvchCtrl_B_HpcPtcEnad/1 -> Switch2/2
  Saturation2/1 -> NegAndPosCheck 5/1(SetPoint), Add2/2
  Add2/1 -> NegAndPosCheck 4/1(SetPoint)
  Unary Minus/1 -> rTmComprCtrl_Te_s32TempError/1

== system ScriptDemo/Create/createMerge/After/SM6/SM6FFEnable ==
  xTmComprCtrl_B_CompOnReqCompOn : Inport  OutDataTypeStr=boolean
  Compare To Constant2 : simulink/Logic and Bit Operations/Compare To Constant  relop===  const=0  OutDataTypeStr=boolean
  Compare To Constant3 : simulink/Logic and Bit Operations/Compare To Constant  relop===  const=1  OutDataTypeStr=boolean
  Logical Operator3 : Logic  AllPortsSameDT=off  OutDataTypeStr=boolean
  PeriodTrig : Subsystem  mask{CounterLim=cTmComprCtrl_t_u16SM6CmpHeatFFPeriod}
      mask DialogControl ParameterGroupVar Prompt: 参数
  Unit Delay : UnitDelay  SampleTime=-1  HasFrameUpgradeWarning=on
  SM6FFEnable_B_SM6FFEnable : Outport  OutDataTypeStr=boolean
  wires:
  Unit Delay/1 -> Compare To Constant2/1
  [xTmComprCtrl_B_CompOnReqCompOn] -> Compare To Constant3/1, Unit Delay/1
  Compare To Constant2/1 -> Logical Operator3/1
  Logical Operator3/1 -> PeriodTrig/1(Counter_Reset)
  Compare To Constant3/1 -> Logical Operator3/2
  xTmComprCtrl_B_CompOnReqCompOn/1 -> [xTmComprCtrl_B_CompOnReqCompOn]
  PeriodTrig/1(Counter_Trig) -> SM6FFEnable_B_SM6FFEnable/1

== system ScriptDemo/Create/createMerge/After/SM6/SM6_Ki ==
  sTmComprCtrl_D_u8HvacFlowLevel : Inport  OutDataTypeStr=uint8
  rTmComprCtrl_Te_s32TempError : Inport  Port=2
  Flow2Rpm : Subsystem  mask{BlwHeatLevel_db=cTmComprCtrl_D_u8HvacFlowTable_db, BlwHeatLevel_sw=cTmComprCtrl_D_u8HvacFlowTable_sw, FFBlw1=mTmComprCtrl_n_u16KiSM6CompHeatRpm_Flow1, FFBlw1_Y=mTmComprCtrl_n_u16KiSM6CompHeatRpm_Flow1_Y, FFBlw1_X=mTmComprCtrl_n_u16KiSM6CompHeatRpm_Flow1_X, FFBlw3=mTmComprCtrl_n_u16KiSM6CompHeatRpm_Flow3, FFBlw3_Y=mTmComprCtrl_n_u16KiSM6CompHeatRpm_Flow3_Y, FFBlw3_X=mTmComprCtrl_n_u16KiSM6CompHeatRpm_Flow3_X, FFBlw5=mTmComprCtrl_n_u16KiSM6CompHeatRpm_Flow5, FFBlw5_Y=mTmComprCtrl_n_u16KiSM6CompHeatRpm_Flow5_Y, FFBlw5_X=mTmComprCtrl_n_u16KiSM6CompHeatRpm_Flow5_X, FFBlw7=mTmComprCtrl_n_u16KiSM6CompHeatRpm_Flow7, FFBlw7_Y=mTmComprCtrl_n_u16KiSM6CompHeatRpm_Flow7_Y, FFBlw7_X=mTmComprCtrl_n_u16KiSM6CompHeatRpm_Flow7_X, FFBlw9=mTmComprCtrl_n_u16KiSM6CompHeatRpm_Flow9, FFBlw9_Y=mTmComprCtrl_n_u16KiSM6CompHeatRpm_Flow9_Y, FFBlw9_X=mTmComprCtrl_n_u16KiSM6CompHeatRpm_Flow9_X}
      mask DialogControl ParameterGroupVar Prompt: 参数
  SM6Ki : Outport
  wires:
  Flow2Rpm/1(Flow2Rpm) -> SM6Ki/1
  ? -> Flow2Rpm/2(breakpoint1)
  sTmComprCtrl_D_u8HvacFlowLevel/1 -> Flow2Rpm/1(md_u8Blw)
  rTmComprCtrl_Te_s32TempError/1 -> Flow2Rpm/3(breakpoint2)

== system ScriptDemo/Create/createMerge/After/SM6/SM6_Kp ==
  sTmComprCtrl_D_u8HvacFlowLevel : Inport  OutDataTypeStr=uint8
  rTmComprCtrl_Te_s32TempError : Inport  Port=2
  Flow2Rpm : Subsystem  mask{BlwHeatLevel_db=cTmComprCtrl_D_u8HvacFlowTable_db, BlwHeatLevel_sw=cTmComprCtrl_D_u8HvacFlowTable_sw, FFBlw1=mTmComprCtrl_n_u16KpSM6CompHeatRpm_Flow1, FFBlw1_Y=mTmComprCtrl_n_u16KpSM6CompHeatRpm_Flow1_Y, FFBlw1_X=mTmComprCtrl_n_u16KpSM6CompHeatRpm_Flow1_X, FFBlw3=mTmComprCtrl_n_u16KpSM6CompHeatRpm_Flow3, FFBlw3_Y=mTmComprCtrl_n_u16KpSM6CompHeatRpm_Flow3_Y, FFBlw3_X=mTmComprCtrl_n_u16KpSM6CompHeatRpm_Flow3_X, FFBlw5=mTmComprCtrl_n_u16KpSM6CompHeatRpm_Flow5, FFBlw5_Y=mTmComprCtrl_n_u16KpSM6CompHeatRpm_Flow5_Y, FFBlw5_X=mTmComprCtrl_n_u16KpSM6CompHeatRpm_Flow5_X, FFBlw7=mTmComprCtrl_n_u16KpSM6CompHeatRpm_Flow7, FFBlw7_Y=mTmComprCtrl_n_u16KpSM6CompHeatRpm_Flow7_Y, FFBlw7_X=mTmComprCtrl_n_u16KpSM6CompHeatRpm_Flow7_X, FFBlw9=mTmComprCtrl_n_u16KpSM6CompHeatRpm_Flow9, FFBlw9_Y=mTmComprCtrl_n_u16KpSM6CompHeatRpm_Flow9_Y, FFBlw9_X=mTmComprCtrl_n_u16KpSM6CompHeatRpm_Flow9_X}
      mask DialogControl ParameterGroupVar Prompt: 参数
  SM6Kp : Outport
  wires:
  Flow2Rpm/1(Flow2Rpm) -> SM6Kp/1
  sTmComprCtrl_D_u8HvacFlowLevel/1 -> Flow2Rpm/1(md_u8Blw)
  ? -> Flow2Rpm/2(breakpoint1)
  rTmComprCtrl_Te_s32TempError/1 -> Flow2Rpm/3(breakpoint2)

== system ScriptDemo/Create/createMerge/Before/ID29332_RpmPI/ClearInteg ==
  rPIControler_n_s32SAccmKi : Inport  OutDataTypeStr=single
  sTmSigProces_Te_s32EvapFanFilter : Inport  Port=2  OutDataTypeStr=single
  xTmComprCtrl_B_CompOnReqCompOn : Inport  Port=3  OutDataTypeStr=boolean
  xTmComprCtrl_B_ModeChanged : Inport  Port=4  OutDataTypeStr=boolean
  yTmRefriModeMgr_B_HeatModeInCycle : Inport  Port=5  OutDataTypeStr=boolean
  Compare To Constant : simulink/Logic and Bit Operations/Compare To Constant  relop===  const=0  OutDataTypeStr=boolean
  Compare To Constant1 : simulink/Logic and Bit Operations/Compare To Constant  relop=>  const=0  OutDataTypeStr=boolean
  Compare To Constant2 : simulink/Logic and Bit Operations/Compare To Constant  relop===  const=[2 22]  OutDataTypeStr=boolean
  Compare To Constant3 : simulink/Logic and Bit Operations/Compare To Constant  relop=<=  const=cTmComprCtrl_Te_EvapClearInteg  OutDataTypeStr=boolean
  Logical Operator : Logic  Operator=OR  Inputs=4  AllPortsSameDT=off  OutDataTypeStr=boolean
  Logical Operator1 : Logic  Inputs=3  AllPortsSameDT=off  OutDataTypeStr=boolean
  Logical Operator2 : Logic  Operator=OR  Inputs=1  AllPortsSameDT=off  OutDataTypeStr=boolean
  Logical Operator3 : Logic  Operator=OR  AllPortsSameDT=off  OutDataTypeStr=boolean
  Unit Delay : UnitDelay  SampleTime=-1  HasFrameUpgradeWarning=on
  xClearInteg_B_ClearInteg : Outport  OutDataTypeStr=boolean
  wires:
  [xTmComprCtrl_B_ModeChanged] -> Logical Operator/2
  Compare To Constant/1 -> Logical Operator/1
  [xTmComprCtrl_B_CompOnReqCompOn] -> Compare To Constant/1
  Logical Operator/1 -> [xTmComprCtrl_B_ClearInteg]  "xTmComprCtrl_B_ClearInteg"
  [rPIControler_n_s32SAccmKi] -> Unit Delay/1
  [sTmRefriModeMgr_D_u8HPCurMode] -> Compare To Constant2/1
  [sTmSigProces_Te_s32EvapFanFilter] -> Compare To Constant3/1
  Compare To Constant2/1 -> Logical Operator2/1
  Compare To Constant1/1 -> Logical Operator1/1
  Compare To Constant3/1 -> Logical Operator1/3
  Logical Operator1/1 -> Logical Operator/3
  rPIControler_n_s32SAccmKi/1 -> [rPIControler_n_s32SAccmKi]
  ? -> [sTmRefriModeMgr_D_u8HPCurMode]
  sTmSigProces_Te_s32EvapFanFilter/1 -> [sTmSigProces_Te_s32EvapFanFilter]
  xTmComprCtrl_B_CompOnReqCompOn/1 -> [xTmComprCtrl_B_CompOnReqCompOn]
  xTmComprCtrl_B_ModeChanged/1 -> [xTmComprCtrl_B_ModeChanged]
  [xTmComprCtrl_B_ClearInteg] -> xClearInteg_B_ClearInteg/1
  Unit Delay/1 -> Compare To Constant1/1
  Logical Operator2/1 -> Logical Operator1/2
  [yTmRefriModeMgr_B_CoolModeInCycle] -> Logical Operator3/1
  [yTmRefriModeMgr_B_HeatModeInCycle] -> Logical Operator3/2
  Logical Operator3/1 -> Logical Operator/4
  ? -> [yTmRefriModeMgr_B_CoolModeInCycle]
  yTmRefriModeMgr_B_HeatModeInCycle/1 -> [yTmRefriModeMgr_B_HeatModeInCycle]
